simulink model "sine_pwm_inverter"  (R2023b)
settings: Solver=VariableStepAuto  StartTime=0.0  StopTime=2  RelTol=1e-3
libraries: spsIGBTDiodeLib x6, spsSeriesRLCBranchLib x6, spsDCVoltageSourceLib x2, spsGroundLib x2, spsMultimeterLib x1, spsSawtoothGeneratorLib x1, spspowerguiLib x1
settings Model: Creator=lmanglicmot  LastModifiedBy=lmanglicmot
settings DataIOCC: ReturnWorkspaceOutputs=off
settings OptimizationCC: ReuseModelBlockBuffer=off

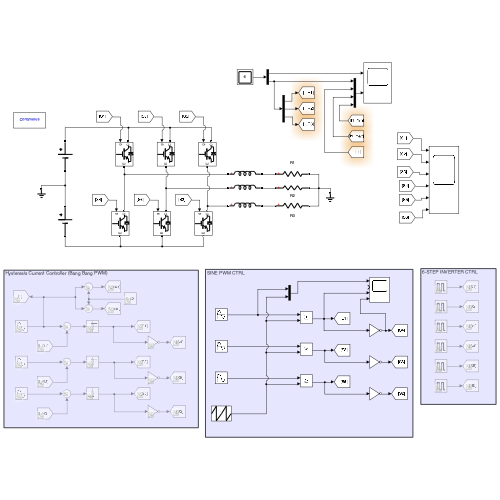
[thumbnail: Simulink's stored preview of the top-level diagram]
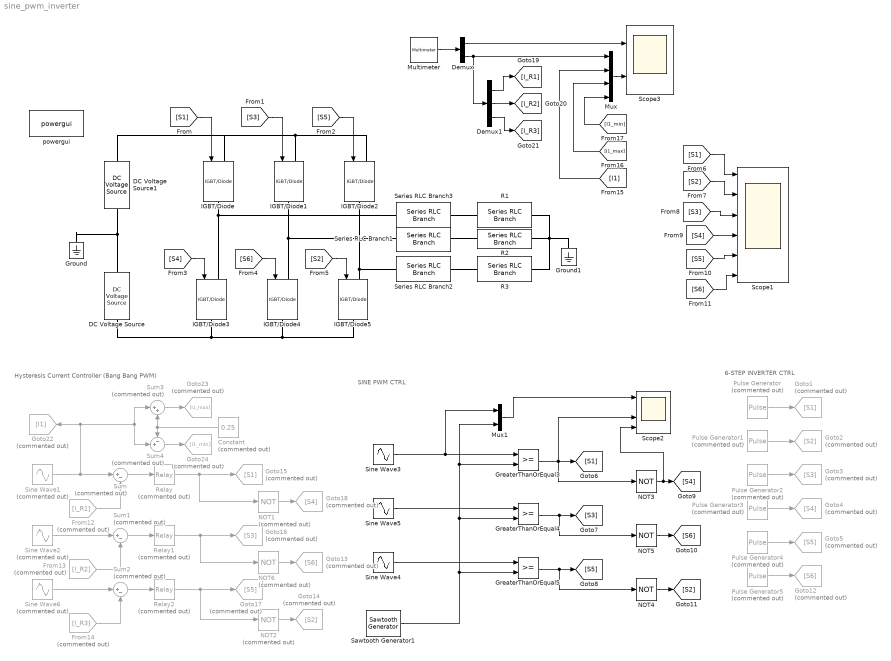
== system sine_pwm_inverter ==
  note: Hysteresis Current Controller (Bang Bang PWM)
  note: SINE PWM CTRL
  note: 6-STEP INVERTER CTRL
  Constant : Constant  Commented=on  Value=0.25
  DC Voltage Source : spsDCVoltageSourceLib/DC Voltage Source  Amplitude=50  Measurements=None
  DC Voltage Source1 : spsDCVoltageSourceLib/DC Voltage Source  Amplitude=50  Measurements=None
  Demux : Demux  Outputs=2
  Demux1 : Demux  Outputs=3
  From12 : From  Commented=on  GotoTag=I_R1
  From13 : From  Commented=on  GotoTag=I_R2
  From14 : From  Commented=on  GotoTag=I_R3
  Goto1 : Goto  Commented=on  GotoTag=S1
  Goto12 : Goto  Commented=on  GotoTag=S6
  Goto13 : Goto  Commented=on  GotoTag=S6
  Goto14 : Goto  Commented=on  GotoTag=S2
  Goto15 : Goto  Commented=on  GotoTag=S1
  Goto16 : Goto  Commented=on  GotoTag=S3
  Goto17 : Goto  Commented=on  GotoTag=S5
  Goto18 : Goto  Commented=on  GotoTag=S4
  Goto2 : Goto  Commented=on  GotoTag=S2
  Goto22 : Goto  Commented=on  GotoTag=I1
  Goto23 : Goto  Commented=on  GotoTag=I1_max
  Goto24 : Goto  Commented=on  GotoTag=I1_min
  Goto3 : Goto  Commented=on  GotoTag=S3
  Goto4 : Goto  Commented=on  GotoTag=S4
  Goto5 : Goto  Commented=on  GotoTag=S5
  GreaterThanOrEqual3 : RelationalOperator  OutDataTypeStr=boolean  RndMeth=Simplest  InputSameDT=off
  GreaterThanOrEqual4 : RelationalOperator  OutDataTypeStr=boolean  RndMeth=Simplest  InputSameDT=off
  GreaterThanOrEqual5 : RelationalOperator  OutDataTypeStr=boolean  RndMeth=Simplest  InputSameDT=off
  Ground : spsGroundLib/Ground  LConnTagsString=a
  Ground1 : spsGroundLib/Ground  LConnTagsString=a
  IGBT/Diode{,1..5} (6 alike) : spsIGBTDiodeLib/IGBT//Diode  Ron=1e-3  Rs=1e5  Cs=inf  Measurements=off
  Multimeter : spsMultimeterLib/Multimeter  L=9  sel=[1 2 3 7 8 9]  yselected={}  Gain=[1 1 1 1 1 1]  OutputType=Complex  PlotAtSimulationStop=off  PhasorSimulation=off
  Mux : Mux
  Mux1 : Mux  Inputs=2
  NOT1 : Logic  Commented=on  Operator=NOT  IconShape=distinctive  AllPortsSameDT=off  OutDataTypeStr=boolean
  NOT2 : Logic  Commented=on  Operator=NOT  IconShape=distinctive  AllPortsSameDT=off  OutDataTypeStr=boolean
  NOT3 : Logic  Operator=NOT  IconShape=distinctive  AllPortsSameDT=off  OutDataTypeStr=boolean
  NOT4 : Logic  Operator=NOT  IconShape=distinctive  AllPortsSameDT=off  OutDataTypeStr=boolean
  NOT5 : Logic  Operator=NOT  IconShape=distinctive  AllPortsSameDT=off  OutDataTypeStr=boolean
  NOT6 : Logic  Commented=on  Operator=NOT  IconShape=distinctive  AllPortsSameDT=off  OutDataTypeStr=boolean
  Pulse Generator : DiscretePulseGenerator  Commented=on  PulseType=Time based  Period=1/60  PulseWidth=50%
  Pulse Generator1 : DiscretePulseGenerator  Commented=on  PulseType=Time based  Period=1/60  PulseWidth=50%  PhaseDelay=(1/6)*1/60
  Pulse Generator2 : DiscretePulseGenerator  Commented=on  PulseType=Time based  Period=1/60  PulseWidth=50%  PhaseDelay=(2/6)*1/60
  Pulse Generator3 : DiscretePulseGenerator  Commented=on  PulseType=Time based  Period=1/60  PulseWidth=50  PhaseDelay=(3/6)*1/60
  Pulse Generator4 : DiscretePulseGenerator  Commented=on  PulseType=Time based  Period=1/60  PulseWidth=50%  PhaseDelay=(4/6)*1/60
  Pulse Generator5 : DiscretePulseGenerator  Commented=on  PulseType=Time based  Period=1/60  PulseWidth=50%  PhaseDelay=(5/6)*1/60
  R1 : spsSeriesRLCBranchLib/Series RLC Branch  LConnTagsString=__new0  RConnTagsString=__new0  BranchType=R  Resistance=1  Inductance=5  SetiL0=off  InitialCurrent=0  Capacitance=1e-6  Setx0=off  InitialVoltage=0  Measurements=Branch voltage and current
  R2 : spsSeriesRLCBranchLib/Series RLC Branch  LConnTagsString=__new0  RConnTagsString=__new0  BranchType=R  Resistance=1  Inductance=5  SetiL0=off  InitialCurrent=0  Capacitance=1e-6  Setx0=off  InitialVoltage=0  Measurements=Branch voltage and current
  R3 : spsSeriesRLCBranchLib/Series RLC Branch  LConnTagsString=__new0  RConnTagsString=__new0  BranchType=R  Resistance=1  Inductance=5  SetiL0=off  InitialCurrent=0  Capacitance=1e-6  Setx0=off  InitialVoltage=0  Measurements=Branch voltage and current
  Relay : Relay  Commented=on  OnSwitchValue=0.25  OffSwitchValue=-0.25
  Relay1 : Relay  Commented=on  OnSwitchValue=0.25  OffSwitchValue=-0.25
  Relay2 : Relay  Commented=on  OnSwitchValue=0.25  OffSwitchValue=-0.25
  Sawtooth Generator1 : spsSawtoothGeneratorLib/Sawtooth Generator  Freq=60*57  Phase=180  Ts=0
  Scope1 : Scope  NumInputPorts=6
  Scope2 : Scope  NumInputPorts=4
  Scope3 : Scope  NumInputPorts=2
  Series RLC Branch1 : spsSeriesRLCBranchLib/Series RLC Branch  LConnTagsString=__new0  RConnTagsString=__new0  BranchType=L  Resistance=1  Inductance=5e-3  SetiL0=off  InitialCurrent=0  Capacitance=1e-6  Setx0=off  InitialVoltage=0  Measurements=Branch voltage
  Series RLC Branch2 : spsSeriesRLCBranchLib/Series RLC Branch  LConnTagsString=__new0  RConnTagsString=__new0  BranchType=L  Resistance=1  Inductance=5e-3  SetiL0=off  InitialCurrent=0  Capacitance=1e-6  Setx0=off  InitialVoltage=0  Measurements=Branch voltage
  Series RLC Branch3 : spsSeriesRLCBranchLib/Series RLC Branch  LConnTagsString=__new0  RConnTagsString=__new0  BranchType=L  Resistance=1  Inductance=5e-3  SetiL0=off  InitialCurrent=0  Capacitance=1e-6  Setx0=off  InitialVoltage=0  Measurements=Branch voltage
  Sine Wave1 : Sin  Commented=on  Amplitude=25  Frequency=2*pi*60  SampleTime=0
  Sine Wave2 : Sin  Commented=on  Amplitude=25  Frequency=2*pi*60  Phase=2*pi/3  SampleTime=0
  Sine Wave3 : Sin  Frequency=2*pi*60  SampleTime=0
  Sine Wave4 : Sin  Frequency=2*pi*60  Phase=-2*pi/3  SampleTime=0
  Sine Wave5 : Sin  Frequency=2*pi*60  Phase=2*pi/3  SampleTime=0
  Sine Wave6 : Sin  Commented=on  Amplitude=25  Frequency=2*pi*60  Phase=-2*pi/3  SampleTime=0
  Sum : Sum  Commented=on  Inputs=|+-
  Sum1 : Sum  Commented=on  Inputs=|+-
  Sum2 : Sum  Commented=on  Inputs=|+-
  Sum3 : Sum  Commented=on  Inputs=|++
  Sum4 : Sum  Commented=on  Inputs=-+|
  powergui : spspowerguiLib/powergui  Priority=1  SimulationMode=Continuous  SampleTime=1e-6  frequency=60  Iterations=50  frequencyindice=0  Pbase=100e6  ErrMax=1e-4  UnitsV=kV  UnitsW=MW  buscounter=0  FunctionMessages=off  echomessages=off  EnableUseOfTLC=off  CurrentSourceSwitches=off  DisableSnubberDevices=off  DisableRonSwitches=off  DisableVfSwitches=off  DisplayEquations=off  AutomaticDiscreteSolvers=off  SolverType=Tustin/Backward Euler (TBE)  Interpol=off  ExternalGateDelay=off  methode=off  Ts=100  x0status=blocks  SPID=on  SwTol=0  HookPort=off  NonlinearTolerance=1e-4  nMaxIteration=100  ContinueOnMaxIteration=off  RestoreLinks=warning  ResistiveCurrentMeasurement=off  Frange=[0:2:500]  Ylog=off  Xlog=on  ShowGrid=off  save=off  variable=ZData  structure=0  ZoomFFT=off  StartTime=0.0  cycles=1  DisplayStyle=1  fundamental=60  FreqAxis=off  MaxFrequency=1000  frequencyindicesteady=1  RmsSteady=1  display=off
  wires:
  [S1] -> IGBT/Diode/1
  [S3] -> IGBT/Diode1/1
  [S5] -> IGBT/Diode2/1
  [S4] -> IGBT/Diode3/1
  [S6] -> IGBT/Diode4/1
  [S2] -> IGBT/Diode5/1
  GreaterThanOrEqual5/1 -> NOT4/1, [S5]
  NOT3/1 -> Scope2/4, [S4]
  Mux1/1 -> Scope2/1
  NOT4/1 -> [S2]
  GreaterThanOrEqual4/1 -> NOT5/1, [S3]
  GreaterThanOrEqual3/1 -> Scope2/3, [S1], NOT3/1
  NOT5/1 -> [S6]
  Sine Wave3/1 -> Mux1/1, GreaterThanOrEqual3/1
  Sine Wave5/1 -> GreaterThanOrEqual4/1
  Sine Wave4/1 -> GreaterThanOrEqual5/1
  Sawtooth Generator1/1 -> GreaterThanOrEqual5/2, GreaterThanOrEqual4/2, Mux1/2, GreaterThanOrEqual3/2
  Pulse Generator/1 -> Goto1/1
  Pulse Generator1/1 -> Goto2/1
  Pulse Generator2/1 -> Goto3/1
  Pulse Generator3/1 -> Goto4/1
  Pulse Generator4/1 -> Goto5/1
  Pulse Generator5/1 -> Goto12/1
  [S1] -> Scope1/1
  [S2] -> Scope1/2
  [S3] -> Scope1/3
  [S4] -> Scope1/4
  [S5] -> Scope1/5
  [S6] -> Scope1/6
  NOT6/1 -> Goto13/1
  Relay/1 -> NOT1/1, Goto15/1
  Relay1/1 -> Goto16/1, NOT6/1
  NOT2/1 -> Goto14/1
  NOT1/1 -> Goto18/1
  Multimeter/1 -> Demux/1
  Demux/1 -> Scope3/1
  Demux/2 -> Demux1/1, Mux/1
  Demux1/1 -> [I_R1]
  Demux1/2 -> [I_R2]
  Demux1/3 -> [I_R3]
  From12/1 -> Sum/2
  Sum/1 -> Relay/1
  Sum1/1 -> Relay1/1
  From13/1 -> Sum1/2
  Sine Wave2/1 -> Sum1/1
  Sine Wave6/1 -> Sum2/1
  From14/1 -> Sum2/2
  Sum2/1 -> Relay2/1
  Relay2/1 -> NOT2/1, Goto17/1
  Constant/1 -> Sum3/2, Sum4/1
  Sum3/1 -> Goto23/1
  Sum4/1 -> Goto24/1
  Mux/1 -> Scope3/2
  [I1] -> Mux/2
  [I1_max] -> Mux/3
  [I1_min] -> Mux/4
  Sine Wave1/1 -> Goto22/1, Sum3/1, Sum4/2, Sum/1
  connections:
  Series RLC Branch3/LConn1 -- IGBT/Diode/RConn1 -- IGBT/Diode3/LConn1
  IGBT/Diode4/LConn1 -- IGBT/Diode1/RConn1 -- Series RLC Branch1/LConn1
  IGBT/Diode5/LConn1 -- IGBT/Diode2/RConn1 -- Series RLC Branch2/LConn1
  IGBT/Diode/LConn1 -- DC Voltage Source1/RConn1 -- IGBT/Diode2/LConn1 -- IGBT/Diode1/LConn1
  DC Voltage Source/LConn1 -- IGBT/Diode5/RConn1 -- IGBT/Diode4/RConn1 -- IGBT/Diode3/RConn1
  DC Voltage Source/RConn1 -- Ground/LConn1 -- DC Voltage Source1/LConn1
  Series RLC Branch3/RConn1 -- R1/LConn1
  Series RLC Branch1/RConn1 -- R2/LConn1
  Series RLC Branch2/RConn1 -- R3/LConn1
  R1/RConn1 -- Ground1/LConn1 -- R3/RConn1 -- R2/RConn1
